simulink model "example8_7"  (R2020b)
settings: Solver=FixedStepAuto  StartTime=0.0  StopTime=40  RelTol=1e-3
settings Model: Creator=yan  LastModifiedBy=yan

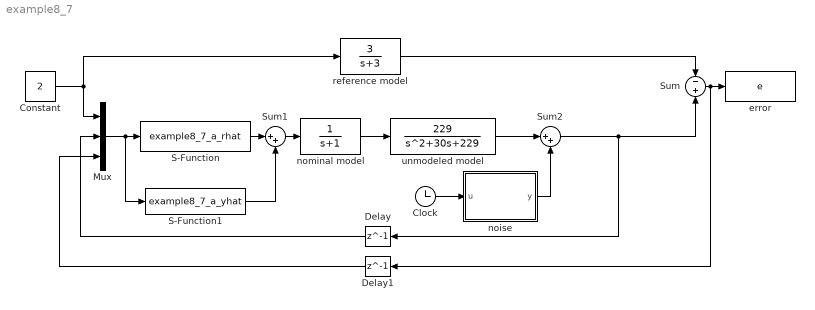
== system example8_7 ==
  Clock : Clock
  Constant : Constant  Value=2
  Delay : Delay  DelayLength=1  InitialCondition=0
  Delay1 : Delay  DelayLength=1  InitialCondition=0
  Mux : Mux  Inputs=3
  S-Function : S-Function  FunctionName=example8_7_a_rhat  SFunctionDeploymentMode=off  EnableBusSupport=off
  S-Function1 : S-Function  FunctionName=example8_7_a_yhat  SFunctionDeploymentMode=off  EnableBusSupport=off
  Sum : Sum  Inputs=-|+
  Sum1 : Sum  Inputs=|++
  Sum2 : Sum  Inputs=|++
  error : ToWorkspace  VariableName=e  SaveFormat=Timeseries  SampleTime=-1
  noise : MATLAB Function  TreatAsAtomicUnit=on
  nominal model : TransferFcn  Denominator=[1 1]
  reference model : TransferFcn  Numerator=[3]  Denominator=[1 3]
  unmodeled model : TransferFcn  Numerator=[229]  Denominator=[1 30 229]
  wires:
  Clock/1 -> noise/1(u)
  S-Function/1 -> Sum1/1
  Sum1/1 -> nominal model/1
  nominal model/1 -> unmodeled model/1
  unmodeled model/1 -> Sum2/1
  Constant/1 -> Mux/1, reference model/1
  noise/1(y) -> Sum2/2
  Sum2/1 -> Delay/1, Sum/2
  reference model/1 -> Sum/1
  S-Function1/1 -> Sum1/2
  Sum/1 -> Delay1/1, error/1
  Mux/1 -> S-Function1/1, S-Function/1
  Delay/1 -> Mux/2
  Delay1/1 -> Mux/3

== matlab function example8_7/noise ==
  data: u input; y output
function y = fcn(u)
y = 0.5*sin(1.61*u);
